simulink model "Modelo_Sim"  (R2015b)
settings: Solver=VariableStepAuto  StartTime=20000  StopTime=40000  RelTol=1e-3
settings Model: Creator=gmiglio  LastModifiedBy=gmiglio

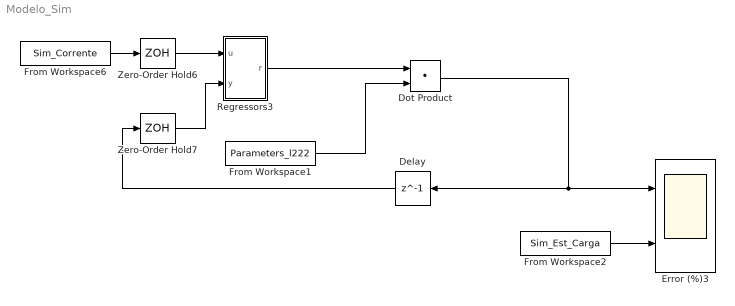
== system Modelo_Sim ==
  Delay : Delay  DelayLength=1  InitialCondition=0  InputProcessing=Inherited  UseCircularBuffer=on  SampleTime=1
  Dot Product : DotProduct  InputSameDT=on  OutDataTypeStr=Inherit: Inherit via internal rule
  Error (%)3 : Scope  NumInputPorts=2
  From Workspace1 : FromWorkspace  VariableName=Parameters_l222  SampleTime=0  Interpolate=off  OutputAfterFinalValue=Holding final value
  From Workspace2 : FromWorkspace  VariableName=Sim_Est_Carga  SampleTime=0
  From Workspace6 : FromWorkspace  VariableName=Sim_Corrente  SampleTime=0
  Regressors3 : Subsystem
  Zero-Order Hold6 : ZeroOrderHold
  Zero-Order Hold7 : ZeroOrderHold
  wires:
  Regressors3/1(r) -> Dot Product/1
  From Workspace6/1 -> Zero-Order Hold6/1
  Delay/1 -> Zero-Order Hold7/1
  Zero-Order Hold6/1 -> Regressors3/1(u)
  Zero-Order Hold7/1 -> Regressors3/2(y)
  From Workspace1/1 -> Dot Product/2
  Dot Product/1 -> Delay/1, Error (%)3/1
  From Workspace2/1 -> Error (%)3/2

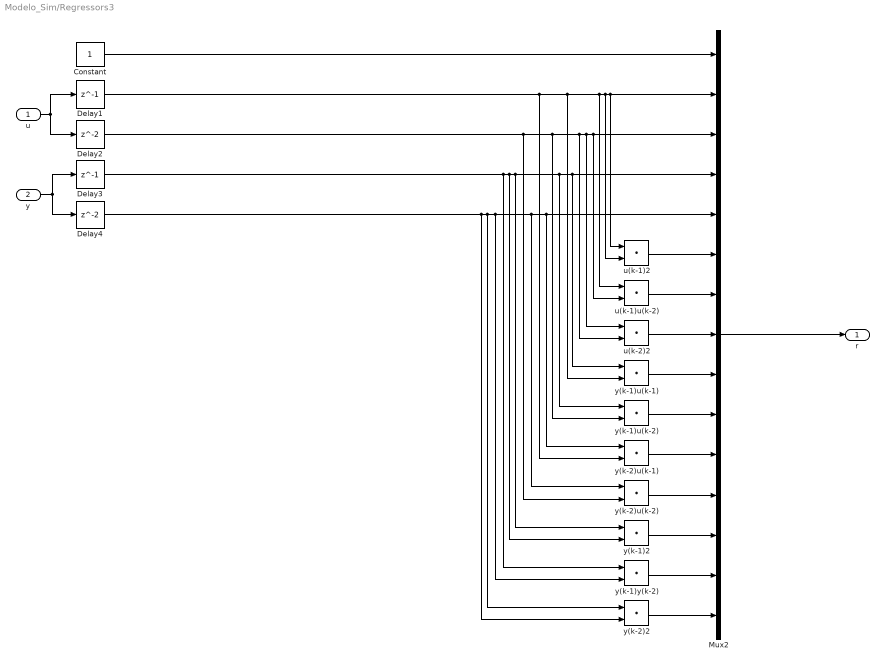
== system Modelo_Sim/Regressors3 ==
  u : Inport
  y : Inport  Port=2
  Constant : Constant
  Delay1 : Delay  DelayLength=1  InitialCondition=0
  Delay2 : Delay  InitialCondition=0
  Delay3 : Delay  DelayLength=1  InitialCondition=0
  Delay4 : Delay  InitialCondition=0
  Mux2 : Mux  Inputs=15
  u(k-1)2 : DotProduct  InputSameDT=on  OutDataTypeStr=Inherit: Inherit via internal rule
  u(k-1)u(k-2) : DotProduct  InputSameDT=on  OutDataTypeStr=Inherit: Inherit via internal rule
  u(k-2)2 : DotProduct  InputSameDT=on  OutDataTypeStr=Inherit: Inherit via internal rule
  y(k-1)2 : DotProduct  InputSameDT=on  OutDataTypeStr=Inherit: Inherit via internal rule
  y(k-1)u(k-1) : DotProduct  InputSameDT=on  OutDataTypeStr=Inherit: Inherit via internal rule
  y(k-1)u(k-2) : DotProduct  InputSameDT=on  OutDataTypeStr=Inherit: Inherit via internal rule
  y(k-1)y(k-2) : DotProduct  InputSameDT=on  OutDataTypeStr=Inherit: Inherit via internal rule
  y(k-2)2 : DotProduct  InputSameDT=on  OutDataTypeStr=Inherit: Inherit via internal rule
  y(k-2)u(k-1) : DotProduct  InputSameDT=on  OutDataTypeStr=Inherit: Inherit via internal rule
  y(k-2)u(k-2) : DotProduct  InputSameDT=on  OutDataTypeStr=Inherit: Inherit via internal rule
  r : Outport
  wires:
  u/1 -> Delay1/1, Delay2/1
  Mux2/1 -> r/1
  Delay1/1 -> y(k-2)u(k-1)/2, y(k-1)u(k-1)/2, u(k-1)u(k-2)/1, u(k-1)2/2, u(k-1)2/1, Mux2/2
  Delay2/1 -> y(k-2)u(k-2)/2, y(k-1)u(k-2)/2, u(k-2)2/2, u(k-2)2/1, u(k-1)u(k-2)/2, Mux2/3
  Constant/1 -> Mux2/1
  u(k-1)2/1 -> Mux2/6
  Delay3/1 -> y(k-1)y(k-2)/1, y(k-1)2/2, y(k-1)2/1, y(k-1)u(k-2)/1, y(k-1)u(k-1)/1, Mux2/4
  Delay4/1 -> y(k-2)2/2, y(k-2)2/1, y(k-1)y(k-2)/2, y(k-2)u(k-2)/1, y(k-2)u(k-1)/1, Mux2/5
  y/1 -> Delay3/1, Delay4/1
  u(k-1)u(k-2)/1 -> Mux2/7
  u(k-2)2/1 -> Mux2/8
  y(k-1)u(k-1)/1 -> Mux2/9
  y(k-1)u(k-2)/1 -> Mux2/10
  y(k-2)u(k-1)/1 -> Mux2/11
  y(k-2)u(k-2)/1 -> Mux2/12
  y(k-1)2/1 -> Mux2/13
  y(k-1)y(k-2)/1 -> Mux2/14
  y(k-2)2/1 -> Mux2/15
